simulink model "testIGRF12"  (Simulink 9.1)
settings: Solver=ode45  StartTime=0.0  StopTime=0  RelTol=1e-3  EnableMultiTasking=on
settings Model: SuppressorTable=22 serialization::archive 11 0 6 0 0 0 0 0  Creator=kikkomi  LastModifiedBy=yyas16  SimulationMode=rapid-accelerator
settings DataIOCC: LimitDataPoints=on
settings DebuggingCC: UnderspecifiedInitializationDetection=Simplified  MergeDetectMultiDrivingBlocksExec=error  SolverPrmCheckMsg=warning
settings GRTTargetCC: GeneratePreprocessorConditionals=Disable all  CombineOutputUpdateFcns=on  GRTInterface=off
settings ConfigComp: CovSFcnEnable=off

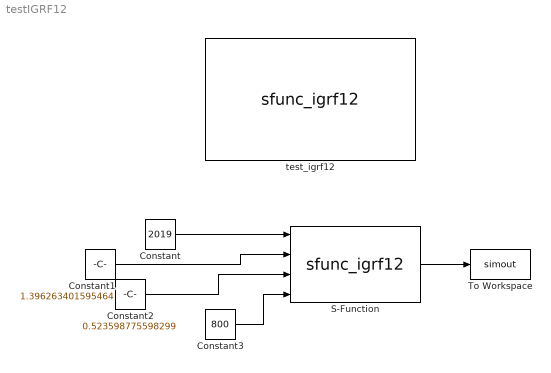
== system testIGRF12 ==
  Constant : Constant  Value=2019
  Constant1 : Constant  Value=1.396263401595464
  Constant2 : Constant  Value=0.523598775598299
  Constant3 : Constant  Value=800
  S-Function : S-Function  FunctionName=sfunc_igrf12  SFunctionDeploymentMode=off  EnableBusSupport=off
  To Workspace : ToWorkspace  VariableName=simout  SampleTime=-1
  test_igrf12 : S-Function  InitFcn=try, set_param(gcb,'FunctionName','sfunc_igrf12'), end  FunctionName=sfunc_igrf12  SFunctionModules=sfunc_igrf12_wrapper igrfsyn12  WizardData=DataTag0  SFunctionDeploymentMode=off  EnableBusSupport=off  mask(S-Function Builder){}
      mask help: Simulink:masks:SFunctionBuilder_MD
      mask init:
      | val = [[.9  0.75 0.75 1 1 .9 .9 1]',[1 1 0.75 0.75 .9 .9 1 .9]'];try , sys = get_param(gcb,'SfunBuilderFcnName');if isempty(sys), sys = get_param(gcb,'FunctionName'); end,catch, sys = get_param(gcb,'FunctionName'); end
      settings: CopyFcn=set_param(gcbh,'LinkStatus','none')  PreSaveFcn=try, set_param(gcb,'FunctionName','sfunc_igrf12'), end  OpenFcn=sfunctionwizard(gcbh)
      mask Display: plot(val(:,1),val(:,2)),disp(sys), port_label('input',1,'fyear'), port_label('input',2,'elon'), port_label('input',3,'nlat'), port_label('input',4,'alt'), port_label('output',1,'b_out')
  wires:
  Constant/1 -> S-Function/1
  Constant1/1 -> S-Function/2
  Constant2/1 -> S-Function/3
  Constant3/1 -> S-Function/4
  S-Function/1 -> To Workspace/1
